simulink model "four_channel_bilateral_teleoperation_architecture_sampled"  (R2020b)
settings: Solver=VariableStepAuto  StartTime=0.0  StopTime=8  RelTol=1e-3
values from neighbouring files (symbols this model uses):
  A = 1    [Assignment_1_continous.m]    (also in Assignment_1_discrete.m = [1 Ts)
  Be = 0    [Assignment_1_continous.m]    (also in Assignment_1_discrete.m)
  Bh = 70    [Assignment_1_continous.m]    (also in Assignment_1_discrete.m)
  Bm = 0.8    [Assignment_1_continous.m]    (also in Assignment_1_discrete.m = 100)
  Bs = 0.8*4    (= 3.2)    [Assignment_1_continous.m]    (also in Assignment_1_discrete.m = 100)
  Dh = 200    [Assignment_1_continous.m]    (also in Assignment_1_discrete.m = 700)
  Dm = 0    [Assignment_1_continous.m]    (also in Assignment_1_discrete.m)
  Ds = 0    [Assignment_1_continous.m]    (also in Assignment_1_discrete.m)
  Fc = 1    [Assignment_1_continous.m]    (also in Assignment_1_discrete.m)
  Fip = 1    [Assignment_1_continous.m]    (also in Assignment_1_discrete.m = 10)
  Je = 0    [Assignment_1_continous.m]    (also in Assignment_1_discrete.m)
  Jh = 0.5    [Assignment_1_continous.m]    (also in Assignment_1_discrete.m = 1)
  Ke = 200    [Assignment_1_continous.m]    (also in Assignment_1_discrete.m)
  Kh = 2000    [Assignment_1_continous.m]    (also in Assignment_1_discrete.m)
  Km = 1    [Assignment_1_continous.m]    (also in Assignment_1_discrete.m = 0)
  Ks = 4    [Assignment_1_continous.m]    (also in Assignment_1_discrete.m = 0)
  Mm = 0.5    [Assignment_1_continous.m]    (also in Assignment_1_discrete.m)
  Ms = 2    [Assignment_1_continous.m]    (also in Assignment_1_discrete.m)
  Ph = 100000    [Assignment_1_continous.m]    (also in Assignment_1_discrete.m = 13000)
  tau = 100000    [Assignment_1_continous.m]    (also in Assignment_1_discrete.m = 10000)
  Ts = 0.001    [Assignment_1_continous.m]    (also in Assignment_1_discrete.m)
libraries: simulink x4
settings Model: Creator=anuj  LastModifiedBy=Edoardo

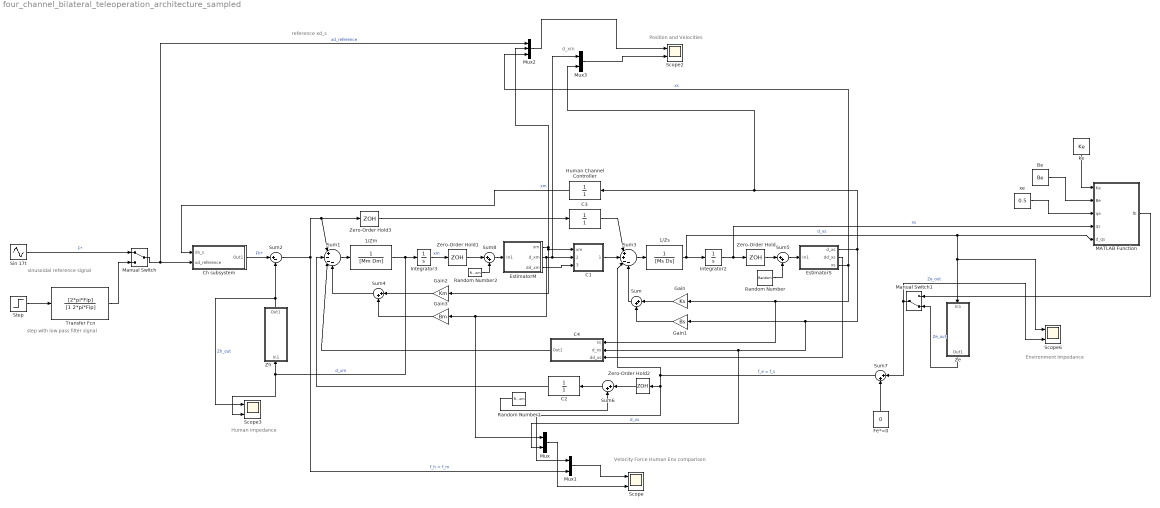
== system four_channel_bilateral_teleoperation_architecture_sampled ==
  note: Position and Velocities
  note: d_xm
  note: reference xd_s
  note: Environment Impedance
  note: Human impedance
  note: Velocity Force Human Env comparison
  note: sinusoidal reference signal
  note: step with low pass filter signal
  1/Zm : TransferFcn  Denominator=[Mm Dm]
  1/Zs : TransferFcn  Denominator=[Ms Ds]
  Be : Constant  Value=Be
  C1 : Subsystem
  C2 : TransferFcn  Denominator=[1]
  C3 : TransferFcn  Denominator=[1]
  C4 : Subsystem
  Ch subsystem : Subsystem
  EstimatorM : Subsystem
  EstimatorS : Subsystem
  Fe*=0 : Constant  Value=0
  Gain : Gain  Gain=Ks
  Gain1 : Gain  Gain=Bs
  Gain2 : Gain  Gain=Km
  Gain3 : Gain  Gain=Bm
  Human Channel Controller : TransferFcn  Denominator=[1]
  Integrator2 : Integrator
  Integrator3 : Integrator
  MATLAB Function : MATLAB Function  TreatAsAtomicUnit=on
  Manual Switch : ManualSwitch
  Manual Switch1 : ManualSwitch  CurrentSetting=0
  Mux : Mux  Inputs=2
  Mux1 : Mux  Inputs=2
  Mux2 : Mux  Inputs=3
  Mux3 : Mux  Inputs=2
  Random Number : RandomNumber  Variance=0.0001  SampleTime=0.1
  Random Number1 : RandomNumber  Variance=0.0001  SampleTime=0.1
  Random Number2 : RandomNumber  Variance=0.0001  SampleTime=0.1
  Scope{,2..3,6} (4 alike) : Scope  NumInputPorts=2
  Sin 17t : Sin  Amplitude=A  Frequency=2*pi*Fc  SampleTime=0
  Step : Step  After=A  SampleTime=0
  Sum{,4..8} (6 alike) : Sum  Inputs=|++
  Sum1 : Sum  Inputs=|+---
  Sum2 : Sum  Inputs=|+-
  Sum3 : Sum  Inputs=|++--
  Transfer Fcn : TransferFcn  Numerator=[2*pi*Fip]  Denominator=[1 2*pi*Fip]
  Ze : Subsystem
  Zero-Order Hold{,1..3} (4 alike) : ZeroOrderHold  SampleTime=Ts
  Zh : Subsystem
  ke : Constant  Value=Ke
  xe : Constant  Value=0.5
  wires:
  Mux/1 -> Scope/2
  Mux1/1 -> Scope/1
  Sum2/1 -> Zero-Order Hold3/1, Sum1/1, Mux1/2  "f_h = f_m"
  1/Zm/1 -> Integrator3/1, Zh/1(In1), Scope3/2  "d_xm"
  Sum1/1 -> 1/Zm/1
  C2/1 -> Sum1/2
  C3/1 -> Sum3/1
  Sum3/1 -> 1/Zs/1
  Fe*=0/1 -> Sum7/2
  Sum7/1 -> Mux1/1, Zero-Order Hold2/1, Sum3/3  "f_e = f_s"
  C4/1(Out1) -> Sum1/3
  Ch subsystem/1(Out1) -> Sum2/1  "Fh*"
  Be/1 -> MATLAB Function/2(Be)
  xe/1 -> MATLAB Function/3(qe)
  ke/1 -> MATLAB Function/1(Ke)
  Integrator2/1 -> Zero-Order Hold/1, MATLAB Function/4(qs)  "xs"
  Transfer Fcn/1 -> Manual Switch/2
  Step/1 -> Transfer Fcn/1
  Human Channel Controller/1 -> Ch subsystem/1(dx_s)
  Manual Switch/1 -> Mux2/1, Ch subsystem/2(xd_reference)  "xd_reference"
  Sin 17t/1 -> Manual Switch/1  "F*"
  C1/1(Out1) -> Sum3/2
  MATLAB Function/1(fE) -> Manual Switch1/1
  1/Zs/1 -> Scope6/1, Ze/1(In1), MATLAB Function/5(d_qs), Integrator2/1  "d_xs"
  Manual Switch1/1 -> Sum7/1, Scope6/2  "Ze_out"
  Zh/1(Out1) -> Sum2/2, Scope3/1  "Zh_out"
  Ze/1(Out1) -> Manual Switch1/2  "Ze_out"
  Mux2/1 -> Scope2/1
  Mux3/1 -> Scope2/2
  Gain/1 -> Sum/1
  Gain1/1 -> Sum/2
  Sum/1 -> Sum3/4
  Sum4/1 -> Sum1/4
  Gain3/1 -> Sum4/2
  Gain2/1 -> Sum4/1
  Integrator3/1 -> Zero-Order Hold1/1  "xm"
  Sum5/1 -> EstimatorS/1(In1)
  Zero-Order Hold/1 -> Sum5/1
  Random Number/1 -> Sum5/2
  Random Number1/1 -> Sum6/2
  Zero-Order Hold2/1 -> Sum6/1
  Sum6/1 -> C2/1
  Zero-Order Hold3/1 -> C3/1
  Random Number2/1 -> Sum8/2
  Zero-Order Hold1/1 -> Sum8/1
  Sum8/1 -> EstimatorM/1(In1)
  EstimatorS/3(xs) -> Mux2/3, C4/1(xs), Gain/1  "xs"
  EstimatorS/1(d_xs) -> Mux3/2, Human Channel Controller/1, C4/2(d_xs), Mux/2, Gain1/1  "d_xs"
  EstimatorS/2(dd_xs) -> C4/3(dd_xs)
  EstimatorM/2(d_xm) -> Mux3/1, C1/2(d_xm), Mux/1, Gain3/1
  EstimatorM/3(dd_xm) -> C1/3(dd_xm)
  EstimatorM/1(xm) -> Gain2/1, C1/1(xm), Mux2/2  "xm"

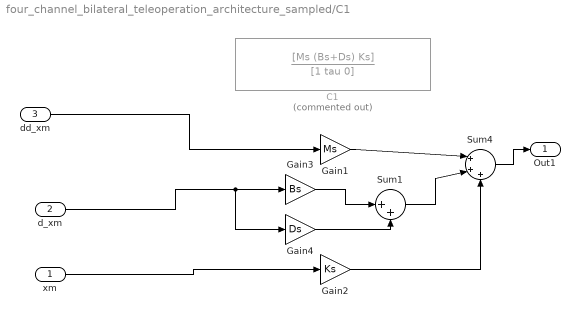
== system four_channel_bilateral_teleoperation_architecture_sampled/C1 ==
  xm : Inport
  d_xm : Inport  Port=2
  dd_xm : Inport  Port=3
  C1 : TransferFcn  Commented=on  Numerator=[Ms (Bs+Ds) Ks]  Denominator=[1 tau 0]
  Gain1 : Gain  Gain=Ms
  Gain2 : Gain  Gain=Ks
  Gain3 : Gain  Gain=Bs
  Gain4 : Gain  Gain=Ds
  Sum1 : Sum  Inputs=|++
  Sum4 : Sum  Inputs=|+++
  Out1 : Outport
  wires:
  Sum4/1 -> Out1/1
  Gain1/1 -> Sum4/1
  Gain2/1 -> Sum4/3
  Sum1/1 -> Sum4/2
  Gain4/1 -> Sum1/2
  Gain3/1 -> Sum1/1
  d_xm/1 -> Gain4/1, Gain3/1
  xm/1 -> Gain2/1
  dd_xm/1 -> Gain1/1

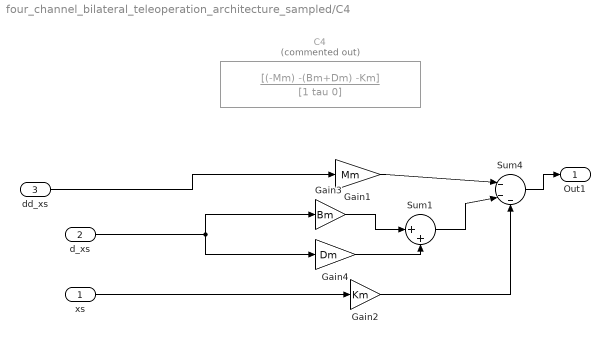
== system four_channel_bilateral_teleoperation_architecture_sampled/C4 ==
  xs : Inport
  d_xs : Inport  Port=2
  dd_xs : Inport  Port=3
  C4 : TransferFcn  Commented=on  Numerator=[(-Mm) -(Bm+Dm) -Km]  Denominator=[1 tau 0]
  Gain1 : Gain  Gain=Mm
  Gain2 : Gain  Gain=Km
  Gain3 : Gain  Gain=Bm
  Gain4 : Gain  Gain=Dm
  Sum1 : Sum  Inputs=|++
  Sum4 : Sum  Inputs=|---
  Out1 : Outport
  wires:
  Sum4/1 -> Out1/1
  Gain1/1 -> Sum4/1
  Gain2/1 -> Sum4/3
  Sum1/1 -> Sum4/2
  Gain4/1 -> Sum1/2
  Gain3/1 -> Sum1/1
  d_xs/1 -> Gain3/1, Gain4/1
  xs/1 -> Gain2/1
  dd_xs/1 -> Gain1/1

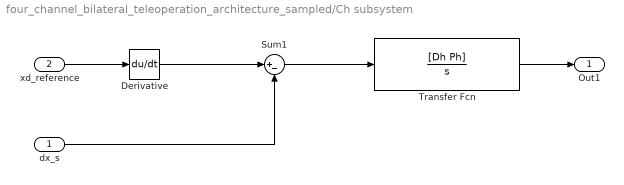
== system four_channel_bilateral_teleoperation_architecture_sampled/Ch subsystem ==
  dx_s : Inport
  xd_reference : Inport  Port=2
  Derivative : Derivative
  Sum1 : Sum  Inputs=|+-
  Transfer Fcn : TransferFcn  Numerator=[Dh Ph]  Denominator=[1 0]
  Out1 : Outport
  wires:
  dx_s/1 -> Sum1/2
  Sum1/1 -> Transfer Fcn/1
  xd_reference/1 -> Derivative/1
  Derivative/1 -> Sum1/1
  Transfer Fcn/1 -> Out1/1

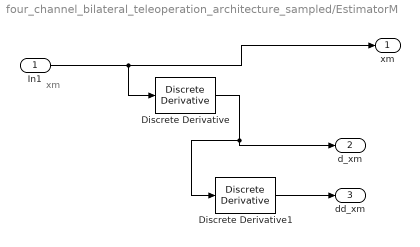
== system four_channel_bilateral_teleoperation_architecture_sampled/EstimatorM ==
  note: xm
  In1 : Inport
  Discrete Derivative : simulink/Discrete/Discrete Derivative  gainval=1.0  ICPrevScaledInput=0.0  OutMin=[]  OutMax=[]  OutDataType=fixdt(1, 16)  OutScaling=2^-10  DoSatur=off
  Discrete Derivative1 : simulink/Discrete/Discrete Derivative  gainval=1.0  ICPrevScaledInput=0.0  OutMin=[]  OutMax=[]  OutDataType=fixdt(1, 16)  OutScaling=2^-10  DoSatur=off
  xm : Outport
  d_xm : Outport  Port=2
  dd_xm : Outport  Port=3
  wires:
  Discrete Derivative/1 -> d_xm/1, Discrete Derivative1/1
  In1/1 -> Discrete Derivative/1, xm/1
  Discrete Derivative1/1 -> dd_xm/1

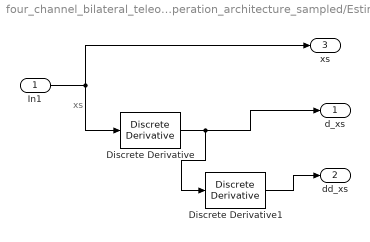
== system four_channel_bilateral_teleoperation_architecture_sampled/EstimatorS ==
  note: xs
  In1 : Inport
  Discrete Derivative : simulink/Discrete/Discrete Derivative  gainval=1.0  ICPrevScaledInput=0.0  OutMin=[]  OutMax=[]  OutDataType=fixdt(1, 16)  OutScaling=2^-10  DoSatur=off
  Discrete Derivative1 : simulink/Discrete/Discrete Derivative  gainval=1.0  ICPrevScaledInput=0.0  OutMin=[]  OutMax=[]  OutDataType=fixdt(1, 16)  OutScaling=2^-10  DoSatur=off
  d_xs : Outport
  dd_xs : Outport  Port=2
  xs : Outport  Port=3
  wires:
  In1/1 -> xs/1, Discrete Derivative/1
  Discrete Derivative/1 -> Discrete Derivative1/1, d_xs/1
  Discrete Derivative1/1 -> dd_xs/1

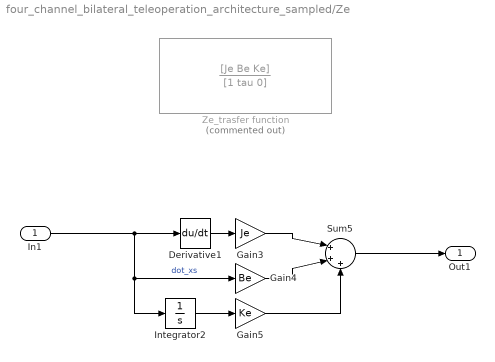
== system four_channel_bilateral_teleoperation_architecture_sampled/Ze ==
  In1 : Inport
  Derivative1 : Derivative
  Gain3 : Gain  Gain=Je
  Gain4 : Gain  Gain=Be
  Gain5 : Gain  Gain=Ke
  Integrator2 : Integrator
  Sum5 : Sum  Inputs=|+++
  Ze_trasfer function : TransferFcn  Commented=on  Numerator=[Je Be Ke]  Denominator=[1 tau 0]
  Out1 : Outport
  wires:
  Gain4/1 -> Sum5/2
  Gain3/1 -> Sum5/1
  Gain5/1 -> Sum5/3
  Sum5/1 -> Out1/1
  Integrator2/1 -> Gain5/1
  In1/1 -> Integrator2/1, Gain4/1, Derivative1/1  "dot_xs"
  Derivative1/1 -> Gain3/1

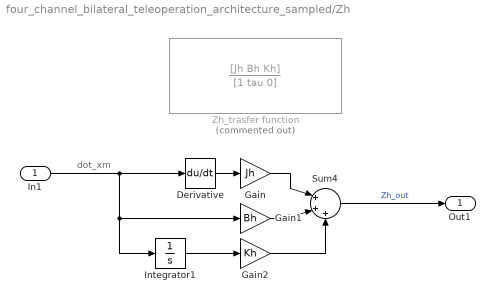
== system four_channel_bilateral_teleoperation_architecture_sampled/Zh ==
  note: dot_xm
  In1 : Inport
  Derivative : Derivative
  Gain : Gain  Gain=Jh
  Gain1 : Gain  Gain=Bh
  Gain2 : Gain  Gain=Kh
  Integrator1 : Integrator
  Sum4 : Sum  Inputs=|+++
  Zh_trasfer function : TransferFcn  Commented=on  Numerator=[Jh Bh Kh]  Denominator=[1 tau 0]
  Out1 : Outport
  wires:
  Derivative/1 -> Gain/1
  Integrator1/1 -> Gain2/1
  Gain2/1 -> Sum4/3
  Gain1/1 -> Sum4/2
  Gain/1 -> Sum4/1
  Sum4/1 -> Out1/1  "Zh_out"
  In1/1 -> Gain1/1, Integrator1/1, Derivative/1

== matlab function four_channel_bilateral_teleoperation_architecture_sampled/MATLAB Function ==
  data: Ke input; fE output; Be input; qe input; qs input; d_qs input
function fE = environment(Ke, Be, qe, qs, d_qs)
    if qs > qe
        fE = Ke * (qs - qe) + Be * qsdot;
    else
        fE = 0;
    end
end
